simulink model "gravcomp"  (Simulink 7.5)
settings: Solver=ode3  StartTime=0.0  StopTime=inf  FixedStep=.002  RelTol=1e-3
undefined symbols (not defined in the file or in its folder): arm_home, arm_j2mt, arm_m2jp, bit, CAN_init, enc_per_rev, fdesignblkfcn, FT_init, gcbh, hand_on, MT_init, puck_I_per_Nm, rotFT2Hand, sample_time, Standard, VL1_init, VL2_init
libraries: simulink x358, xpclib x28, xpcutilitieslib x6, dspmathops x1
(part 3 of 3)

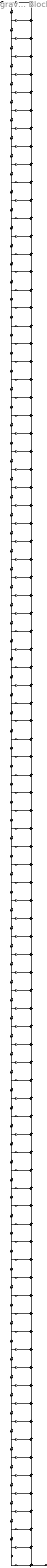
== system gravcomp/Get FT/Get Force Torque/Original Filter/Generated Filter Block ==
  Input : Inport
  BodyDelay{2..88} (87 alike) : simulink/Discrete/Integer Delay  vinit=0  samptime=-1  NumDelays=1
  BodyLSum{2..88} (87 alike) : Sum  Inputs=++|  OutScaling=1  RndMeth=Nearest  SaturateOnIntegerOverflow=on  OutDataTypeStr=Inherit: Same as first input
  b(1) : Gain  Gain=0.00082134311329855878  ParameterDataTypeMode=Specify via dialog  ParameterDataType=float('double')  ParamDataTypeStr=float('double')  OutScaling=1  RndMeth=Nearest  SaturateOnIntegerOverflow=on  OutDataTypeStr=Inherit: Same as input
  b(10) : Gain  Gain=-0.0024150838129607284  ParameterDataTypeMode=Specify via dialog  ParameterDataType=float('double')  ParamDataTypeStr=float('double')  OutScaling=1  RndMeth=Nearest  SaturateOnIntegerOverflow=on  OutDataTypeStr=Inherit: Same as input
  b(11) : Gain  Gain=-0.0039600576183871855  ParameterDataTypeMode=Specify via dialog  ParameterDataType=float('double')  ParamDataTypeStr=float('double')  OutScaling=1  RndMeth=Nearest  SaturateOnIntegerOverflow=on  OutDataTypeStr=Inherit: Same as input
  b(12) : Gain  Gain=-0.0054879111338127914  ParameterDataTypeMode=Specify via dialog  ParameterDataType=float('double')  ParamDataTypeStr=float('double')  OutScaling=1  RndMeth=Nearest  SaturateOnIntegerOverflow=on  OutDataTypeStr=Inherit: Same as input
  b(13) : Gain  Gain=-0.006789571651036521  ParameterDataTypeMode=Specify via dialog  ParameterDataType=float('double')  ParamDataTypeStr=float('double')  OutScaling=1  RndMeth=Nearest  SaturateOnIntegerOverflow=on  OutDataTypeStr=Inherit: Same as input
  b(14) : Gain  Gain=-0.007643017635847205  ParameterDataTypeMode=Specify via dialog  ParameterDataType=float('double')  ParamDataTypeStr=float('double')  OutScaling=1  RndMeth=Nearest  SaturateOnIntegerOverflow=on  OutDataTypeStr=Inherit: Same as input
  b(15) : Gain  Gain=-0.0078436359305586525  ParameterDataTypeMode=Specify via dialog  ParameterDataType=float('double')  ParamDataTypeStr=float('double')  OutScaling=1  RndMeth=Nearest  SaturateOnIntegerOverflow=on  OutDataTypeStr=Inherit: Same as input
  b(16) : Gain  Gain=-0.0072403435516525706  ParameterDataTypeMode=Specify via dialog  ParameterDataType=float('double')  ParamDataTypeStr=float('double')  OutScaling=1  RndMeth=Nearest  SaturateOnIntegerOverflow=on  OutDataTypeStr=Inherit: Same as input
  b(17) : Gain  Gain=-0.0057673738553609957  ParameterDataTypeMode=Specify via dialog  ParameterDataType=float('double')  ParamDataTypeStr=float('double')  OutScaling=1  RndMeth=Nearest  SaturateOnIntegerOverflow=on  OutDataTypeStr=Inherit: Same as input
  b(18) : Gain  Gain=-0.0034717942727364942  ParameterDataTypeMode=Specify via dialog  ParameterDataType=float('double')  ParamDataTypeStr=float('double')  OutScaling=1  RndMeth=Nearest  SaturateOnIntegerOverflow=on  OutDataTypeStr=Inherit: Same as input
  b(19) : Gain  Gain=-0.00052673802500832409  ParameterDataTypeMode=Specify via dialog  ParameterDataType=float('double')  ParamDataTypeStr=float('double')  OutScaling=1  RndMeth=Nearest  SaturateOnIntegerOverflow=on  OutDataTypeStr=Inherit: Same as input
  b(2) : Gain  Gain=0.00086044183774138872  ParameterDataTypeMode=Specify via dialog  ParameterDataType=float('double')  ParamDataTypeStr=float('double')  OutScaling=1  RndMeth=Nearest  SaturateOnIntegerOverflow=on  OutDataTypeStr=Inherit: Same as input
  b(20) : Gain  Gain=0.0027718950549306624  ParameterDataTypeMode=Specify via dialog  ParameterDataType=float('double')  ParamDataTypeStr=float('double')  OutScaling=1  RndMeth=Nearest  SaturateOnIntegerOverflow=on  OutDataTypeStr=Inherit: Same as input
  b(21) : Gain  Gain=0.0060277239934803696  ParameterDataTypeMode=Specify via dialog  ParameterDataType=float('double')  ParamDataTypeStr=float('double')  OutScaling=1  RndMeth=Nearest  SaturateOnIntegerOverflow=on  OutDataTypeStr=Inherit: Same as input
  b(22) : Gain  Gain=0.008783844113631022  ParameterDataTypeMode=Specify via dialog  ParameterDataType=float('double')  ParamDataTypeStr=float('double')  OutScaling=1  RndMeth=Nearest  SaturateOnIntegerOverflow=on  OutDataTypeStr=Inherit: Same as input
  b(23) : Gain  Gain=0.010579384955155813  ParameterDataTypeMode=Specify via dialog  ParameterDataType=float('double')  ParamDataTypeStr=float('double')  OutScaling=1  RndMeth=Nearest  SaturateOnIntegerOverflow=on  OutDataTypeStr=Inherit: Same as input
  b(24) : Gain  Gain=0.011014410167142509  ParameterDataTypeMode=Specify via dialog  ParameterDataType=float('double')  ParamDataTypeStr=float('double')  OutScaling=1  RndMeth=Nearest  SaturateOnIntegerOverflow=on  OutDataTypeStr=Inherit: Same as input
  b(25) : Gain  Gain=0.0098173087600081296  ParameterDataTypeMode=Specify via dialog  ParameterDataType=float('double')  ParamDataTypeStr=float('double')  OutScaling=1  RndMeth=Nearest  SaturateOnIntegerOverflow=on  OutDataTypeStr=Inherit: Same as input
  b(26) : Gain  Gain=0.006903687414337915  ParameterDataTypeMode=Specify via dialog  ParameterDataType=float('double')  ParamDataTypeStr=float('double')  OutScaling=1  RndMeth=Nearest  SaturateOnIntegerOverflow=on  OutDataTypeStr=Inherit: Same as input
  b(27) : Gain  Gain=0.0024180557419036216  ParameterDataTypeMode=Specify via dialog  ParameterDataType=float('double')  ParamDataTypeStr=float('double')  OutScaling=1  RndMeth=Nearest  SaturateOnIntegerOverflow=on  OutDataTypeStr=Inherit: Same as input
  b(28) : Gain  Gain=-0.0032497931384978924  ParameterDataTypeMode=Specify via dialog  ParameterDataType=float('double')  ParamDataTypeStr=float('double')  OutScaling=1  RndMeth=Nearest  SaturateOnIntegerOverflow=on  OutDataTypeStr=Inherit: Same as input
  b(29) : Gain  Gain=-0.0094784288355618199  ParameterDataTypeMode=Specify via dialog  ParameterDataType=float('double')  ParamDataTypeStr=float('double')  OutScaling=1  RndMeth=Nearest  SaturateOnIntegerOverflow=on  OutDataTypeStr=Inherit: Same as input
  b(3) : Gain  Gain=0.0011650777729447837  ParameterDataTypeMode=Specify via dialog  ParameterDataType=float('double')  ParamDataTypeStr=float('double')  OutScaling=1  RndMeth=Nearest  SaturateOnIntegerOverflow=on  OutDataTypeStr=Inherit: Same as input
  b(30) : Gain  Gain=-0.015461211888206202  ParameterDataTypeMode=Specify via dialog  ParameterDataType=float('double')  ParamDataTypeStr=float('double')  OutScaling=1  RndMeth=Nearest  SaturateOnIntegerOverflow=on  OutDataTypeStr=Inherit: Same as input
  b(31) : Gain  Gain=-0.020281532807071435  ParameterDataTypeMode=Specify via dialog  ParameterDataType=float('double')  ParamDataTypeStr=float('double')  OutScaling=1  RndMeth=Nearest  SaturateOnIntegerOverflow=on  OutDataTypeStr=Inherit: Same as input
  b(32) : Gain  Gain=-0.023010985299838312  ParameterDataTypeMode=Specify via dialog  ParameterDataType=float('double')  ParamDataTypeStr=float('double')  OutScaling=1  RndMeth=Nearest  SaturateOnIntegerOverflow=on  OutDataTypeStr=Inherit: Same as input
  b(33) : Gain  Gain=-0.022819440668883396  ParameterDataTypeMode=Specify via dialog  ParameterDataType=float('double')  ParamDataTypeStr=float('double')  OutScaling=1  RndMeth=Nearest  SaturateOnIntegerOverflow=on  OutDataTypeStr=Inherit: Same as input
  b(34) : Gain  Gain=-0.01908434796516191  ParameterDataTypeMode=Specify via dialog  ParameterDataType=float('double')  ParamDataTypeStr=float('double')  OutScaling=1  RndMeth=Nearest  SaturateOnIntegerOverflow=on  OutDataTypeStr=Inherit: Same as input
  b(35) : Gain  Gain=-0.011485203310779294  ParameterDataTypeMode=Specify via dialog  ParameterDataType=float('double')  ParamDataTypeStr=float('double')  OutScaling=1  RndMeth=Nearest  SaturateOnIntegerOverflow=on  OutDataTypeStr=Inherit: Same as input
  b(36) : Gain  Gain=-7.045886460328981e-005  ParameterDataTypeMode=Specify via dialog  ParameterDataType=float('double')  ParamDataTypeStr=float('double')  OutScaling=1  RndMeth=Nearest  SaturateOnIntegerOverflow=on  OutDataTypeStr=Inherit: Same as input
  b(37) : Gain  Gain=0.0147140504913441  ParameterDataTypeMode=Specify via dialog  ParameterDataType=float('double')  ParamDataTypeStr=float('double')  OutScaling=1  RndMeth=Nearest  SaturateOnIntegerOverflow=on  OutDataTypeStr=Inherit: Same as input
  b(38) : Gain  Gain=0.032040450344852957  ParameterDataTypeMode=Specify via dialog  ParameterDataType=float('double')  ParamDataTypeStr=float('double')  OutScaling=1  RndMeth=Nearest  SaturateOnIntegerOverflow=on  OutDataTypeStr=Inherit: Same as input
  b(39) : Gain  Gain=0.050759005066959656  ParameterDataTypeMode=Specify via dialog  ParameterDataType=float('double')  ParamDataTypeStr=float('double')  OutScaling=1  RndMeth=Nearest  SaturateOnIntegerOverflow=on  OutDataTypeStr=Inherit: Same as input
  b(4) : Gain  Gain=0.0013989605197153431  ParameterDataTypeMode=Specify via dialog  ParameterDataType=float('double')  ParamDataTypeStr=float('double')  OutScaling=1  RndMeth=Nearest  SaturateOnIntegerOverflow=on  OutDataTypeStr=Inherit: Same as input
  b(40) : Gain  Gain=0.069498089116120501  ParameterDataTypeMode=Specify via dialog  ParameterDataType=float('double')  ParamDataTypeStr=float('double')  OutScaling=1  RndMeth=Nearest  SaturateOnIntegerOverflow=on  OutDataTypeStr=Inherit: Same as input
  b(41) : Gain  Gain=0.086794001009398575  ParameterDataTypeMode=Specify via dialog  ParameterDataType=float('double')  ParamDataTypeStr=float('double')  OutScaling=1  RndMeth=Nearest  SaturateOnIntegerOverflow=on  OutDataTypeStr=Inherit: Same as input
  b(42) : Gain  Gain=0.10123636540766748  ParameterDataTypeMode=Specify via dialog  ParameterDataType=float('double')  ParamDataTypeStr=float('double')  OutScaling=1  RndMeth=Nearest  SaturateOnIntegerOverflow=on  OutDataTypeStr=Inherit: Same as input
  b(43) : Gain  Gain=0.11161274108764474  ParameterDataTypeMode=Specify via dialog  ParameterDataType=float('double')  ParamDataTypeStr=float('double')  OutScaling=1  RndMeth=Nearest  SaturateOnIntegerOverflow=on  OutDataTypeStr=Inherit: Same as input
  b(44) : Gain  Gain=0.11703538988284418  ParameterDataTypeMode=Specify via dialog  ParameterDataType=float('double')  ParamDataTypeStr=float('double')  OutScaling=1  RndMeth=Nearest  SaturateOnIntegerOverflow=on  OutDataTypeStr=Inherit: Same as input
  b(45) : Gain  Gain=0.11703538988284418  ParameterDataTypeMode=Specify via dialog  ParameterDataType=float('double')  ParamDataTypeStr=float('double')  OutScaling=1  RndMeth=Nearest  SaturateOnIntegerOverflow=on  OutDataTypeStr=Inherit: Same as input
  b(46) : Gain  Gain=0.11161274108764474  ParameterDataTypeMode=Specify via dialog  ParameterDataType=float('double')  ParamDataTypeStr=float('double')  OutScaling=1  RndMeth=Nearest  SaturateOnIntegerOverflow=on  OutDataTypeStr=Inherit: Same as input
  b(47) : Gain  Gain=0.10123636540766748  ParameterDataTypeMode=Specify via dialog  ParameterDataType=float('double')  ParamDataTypeStr=float('double')  OutScaling=1  RndMeth=Nearest  SaturateOnIntegerOverflow=on  OutDataTypeStr=Inherit: Same as input
  b(48) : Gain  Gain=0.086794001009398575  ParameterDataTypeMode=Specify via dialog  ParameterDataType=float('double')  ParamDataTypeStr=float('double')  OutScaling=1  RndMeth=Nearest  SaturateOnIntegerOverflow=on  OutDataTypeStr=Inherit: Same as input
  b(49) : Gain  Gain=0.069498089116120501  ParameterDataTypeMode=Specify via dialog  ParameterDataType=float('double')  ParamDataTypeStr=float('double')  OutScaling=1  RndMeth=Nearest  SaturateOnIntegerOverflow=on  OutDataTypeStr=Inherit: Same as input
  b(5) : Gain  Gain=0.0014807379825975565  ParameterDataTypeMode=Specify via dialog  ParameterDataType=float('double')  ParamDataTypeStr=float('double')  OutScaling=1  RndMeth=Nearest  SaturateOnIntegerOverflow=on  OutDataTypeStr=Inherit: Same as input
  b(50) : Gain  Gain=0.050759005066959656  ParameterDataTypeMode=Specify via dialog  ParameterDataType=float('double')  ParamDataTypeStr=float('double')  OutScaling=1  RndMeth=Nearest  SaturateOnIntegerOverflow=on  OutDataTypeStr=Inherit: Same as input
  b(51) : Gain  Gain=0.032040450344852957  ParameterDataTypeMode=Specify via dialog  ParameterDataType=float('double')  ParamDataTypeStr=float('double')  OutScaling=1  RndMeth=Nearest  SaturateOnIntegerOverflow=on  OutDataTypeStr=Inherit: Same as input
  b(52) : Gain  Gain=0.0147140504913441  ParameterDataTypeMode=Specify via dialog  ParameterDataType=float('double')  ParamDataTypeStr=float('double')  OutScaling=1  RndMeth=Nearest  SaturateOnIntegerOverflow=on  OutDataTypeStr=Inherit: Same as input
  b(53) : Gain  Gain=-7.045886460328981e-005  ParameterDataTypeMode=Specify via dialog  ParameterDataType=float('double')  ParamDataTypeStr=float('double')  OutScaling=1  RndMeth=Nearest  SaturateOnIntegerOverflow=on  OutDataTypeStr=Inherit: Same as input
  b(54) : Gain  Gain=-0.011485203310779294  ParameterDataTypeMode=Specify via dialog  ParameterDataType=float('double')  ParamDataTypeStr=float('double')  OutScaling=1  RndMeth=Nearest  SaturateOnIntegerOverflow=on  OutDataTypeStr=Inherit: Same as input
  b(55) : Gain  Gain=-0.01908434796516191  ParameterDataTypeMode=Specify via dialog  ParameterDataType=float('double')  ParamDataTypeStr=float('double')  OutScaling=1  RndMeth=Nearest  SaturateOnIntegerOverflow=on  OutDataTypeStr=Inherit: Same as input
  b(56) : Gain  Gain=-0.022819440668883396  ParameterDataTypeMode=Specify via dialog  ParameterDataType=float('double')  ParamDataTypeStr=float('double')  OutScaling=1  RndMeth=Nearest  SaturateOnIntegerOverflow=on  OutDataTypeStr=Inherit: Same as input
  b(57) : Gain  Gain=-0.023010985299838312  ParameterDataTypeMode=Specify via dialog  ParameterDataType=float('double')  ParamDataTypeStr=float('double')  OutScaling=1  RndMeth=Nearest  SaturateOnIntegerOverflow=on  OutDataTypeStr=Inherit: Same as input
  b(58) : Gain  Gain=-0.020281532807071435  ParameterDataTypeMode=Specify via dialog  ParameterDataType=float('double')  ParamDataTypeStr=float('double')  OutScaling=1  RndMeth=Nearest  SaturateOnIntegerOverflow=on  OutDataTypeStr=Inherit: Same as input
  b(59) : Gain  Gain=-0.015461211888206202  ParameterDataTypeMode=Specify via dialog  ParameterDataType=float('double')  ParamDataTypeStr=float('double')  OutScaling=1  RndMeth=Nearest  SaturateOnIntegerOverflow=on  OutDataTypeStr=Inherit: Same as input
  b(6) : Gain  Gain=0.0013305171923252142  ParameterDataTypeMode=Specify via dialog  ParameterDataType=float('double')  ParamDataTypeStr=float('double')  OutScaling=1  RndMeth=Nearest  SaturateOnIntegerOverflow=on  OutDataTypeStr=Inherit: Same as input
  b(60) : Gain  Gain=-0.0094784288355618199  ParameterDataTypeMode=Specify via dialog  ParameterDataType=float('double')  ParamDataTypeStr=float('double')  OutScaling=1  RndMeth=Nearest  SaturateOnIntegerOverflow=on  OutDataTypeStr=Inherit: Same as input
  b(61) : Gain  Gain=-0.0032497931384978924  ParameterDataTypeMode=Specify via dialog  ParameterDataType=float('double')  ParamDataTypeStr=float('double')  OutScaling=1  RndMeth=Nearest  SaturateOnIntegerOverflow=on  OutDataTypeStr=Inherit: Same as input
  b(62) : Gain  Gain=0.0024180557419036216  ParameterDataTypeMode=Specify via dialog  ParameterDataType=float('double')  ParamDataTypeStr=float('double')  OutScaling=1  RndMeth=Nearest  SaturateOnIntegerOverflow=on  OutDataTypeStr=Inherit: Same as input
  b(63) : Gain  Gain=0.006903687414337915  ParameterDataTypeMode=Specify via dialog  ParameterDataType=float('double')  ParamDataTypeStr=float('double')  OutScaling=1  RndMeth=Nearest  SaturateOnIntegerOverflow=on  OutDataTypeStr=Inherit: Same as input
  b(64) : Gain  Gain=0.0098173087600081296  ParameterDataTypeMode=Specify via dialog  ParameterDataType=float('double')  ParamDataTypeStr=float('double')  OutScaling=1  RndMeth=Nearest  SaturateOnIntegerOverflow=on  OutDataTypeStr=Inherit: Same as input
  b(65) : Gain  Gain=0.011014410167142509  ParameterDataTypeMode=Specify via dialog  ParameterDataType=float('double')  ParamDataTypeStr=float('double')  OutScaling=1  RndMeth=Nearest  SaturateOnIntegerOverflow=on  OutDataTypeStr=Inherit: Same as input
  b(66) : Gain  Gain=0.010579384955155813  ParameterDataTypeMode=Specify via dialog  ParameterDataType=float('double')  ParamDataTypeStr=float('double')  OutScaling=1  RndMeth=Nearest  SaturateOnIntegerOverflow=on  OutDataTypeStr=Inherit: Same as input
  b(67) : Gain  Gain=0.008783844113631022  ParameterDataTypeMode=Specify via dialog  ParameterDataType=float('double')  ParamDataTypeStr=float('double')  OutScaling=1  RndMeth=Nearest  SaturateOnIntegerOverflow=on  OutDataTypeStr=Inherit: Same as input
  b(68) : Gain  Gain=0.0060277239934803696  ParameterDataTypeMode=Specify via dialog  ParameterDataType=float('double')  ParamDataTypeStr=float('double')  OutScaling=1  RndMeth=Nearest  SaturateOnIntegerOverflow=on  OutDataTypeStr=Inherit: Same as input
  b(69) : Gain  Gain=0.0027718950549306624  ParameterDataTypeMode=Specify via dialog  ParameterDataType=float('double')  ParamDataTypeStr=float('double')  OutScaling=1  RndMeth=Nearest  SaturateOnIntegerOverflow=on  OutDataTypeStr=Inherit: Same as input
  b(7) : Gain  Gain=0.0008813799288182459  ParameterDataTypeMode=Specify via dialog  ParameterDataType=float('double')  ParamDataTypeStr=float('double')  OutScaling=1  RndMeth=Nearest  SaturateOnIntegerOverflow=on  OutDataTypeStr=Inherit: Same as input
  b(70) : Gain  Gain=-0.00052673802500832409  ParameterDataTypeMode=Specify via dialog  ParameterDataType=float('double')  ParamDataTypeStr=float('double')  OutScaling=1  RndMeth=Nearest  SaturateOnIntegerOverflow=on  OutDataTypeStr=Inherit: Same as input
  b(71) : Gain  Gain=-0.0034717942727364942  ParameterDataTypeMode=Specify via dialog  ParameterDataType=float('double')  ParamDataTypeStr=float('double')  OutScaling=1  RndMeth=Nearest  SaturateOnIntegerOverflow=on  OutDataTypeStr=Inherit: Same as input
  b(72) : Gain  Gain=-0.0057673738553609957  ParameterDataTypeMode=Specify via dialog  ParameterDataType=float('double')  ParamDataTypeStr=float('double')  OutScaling=1  RndMeth=Nearest  SaturateOnIntegerOverflow=on  OutDataTypeStr=Inherit: Same as input
  b(73) : Gain  Gain=-0.0072403435516525706  ParameterDataTypeMode=Specify via dialog  ParameterDataType=float('double')  ParamDataTypeStr=float('double')  OutScaling=1  RndMeth=Nearest  SaturateOnIntegerOverflow=on  OutDataTypeStr=Inherit: Same as input
  b(74) : Gain  Gain=-0.0078436359305586525  ParameterDataTypeMode=Specify via dialog  ParameterDataType=float('double')  ParamDataTypeStr=float('double')  OutScaling=1  RndMeth=Nearest  SaturateOnIntegerOverflow=on  OutDataTypeStr=Inherit: Same as input
  b(75) : Gain  Gain=-0.007643017635847205  ParameterDataTypeMode=Specify via dialog  ParameterDataType=float('double')  ParamDataTypeStr=float('double')  OutScaling=1  RndMeth=Nearest  SaturateOnIntegerOverflow=on  OutDataTypeStr=Inherit: Same as input
  b(76) : Gain  Gain=-0.006789571651036521  ParameterDataTypeMode=Specify via dialog  ParameterDataType=float('double')  ParamDataTypeStr=float('double')  OutScaling=1  RndMeth=Nearest  SaturateOnIntegerOverflow=on  OutDataTypeStr=Inherit: Same as input
  b(77) : Gain  Gain=-0.0054879111338127914  ParameterDataTypeMode=Specify via dialog  ParameterDataType=float('double')  ParamDataTypeStr=float('double')  OutScaling=1  RndMeth=Nearest  SaturateOnIntegerOverflow=on  OutDataTypeStr=Inherit: Same as input
  b(78) : Gain  Gain=-0.0039600576183871855  ParameterDataTypeMode=Specify via dialog  ParameterDataType=float('double')  ParamDataTypeStr=float('double')  OutScaling=1  RndMeth=Nearest  SaturateOnIntegerOverflow=on  OutDataTypeStr=Inherit: Same as input
  b(79) : Gain  Gain=-0.0024150838129607284  ParameterDataTypeMode=Specify via dialog  ParameterDataType=float('double')  ParamDataTypeStr=float('double')  OutScaling=1  RndMeth=Nearest  SaturateOnIntegerOverflow=on  OutDataTypeStr=Inherit: Same as input
  b(8) : Gain  Gain=9.3966665944649592e-005  ParameterDataTypeMode=Specify via dialog  ParameterDataType=float('double')  ParamDataTypeStr=float('double')  OutScaling=1  RndMeth=Nearest  SaturateOnIntegerOverflow=on  OutDataTypeStr=Inherit: Same as input
  b(80) : Gain  Gain=-0.0010242764933667812  ParameterDataTypeMode=Specify via dialog  ParameterDataType=float('double')  ParamDataTypeStr=float('double')  OutScaling=1  RndMeth=Nearest  SaturateOnIntegerOverflow=on  OutDataTypeStr=Inherit: Same as input
  b(81) : Gain  Gain=9.3966665944649592e-005  ParameterDataTypeMode=Specify via dialog  ParameterDataType=float('double')  ParamDataTypeStr=float('double')  OutScaling=1  RndMeth=Nearest  SaturateOnIntegerOverflow=on  OutDataTypeStr=Inherit: Same as input
  b(82) : Gain  Gain=0.0008813799288182459  ParameterDataTypeMode=Specify via dialog  ParameterDataType=float('double')  ParamDataTypeStr=float('double')  OutScaling=1  RndMeth=Nearest  SaturateOnIntegerOverflow=on  OutDataTypeStr=Inherit: Same as input
  b(83) : Gain  Gain=0.0013305171923252142  ParameterDataTypeMode=Specify via dialog  ParameterDataType=float('double')  ParamDataTypeStr=float('double')  OutScaling=1  RndMeth=Nearest  SaturateOnIntegerOverflow=on  OutDataTypeStr=Inherit: Same as input
  b(84) : Gain  Gain=0.0014807379825975565  ParameterDataTypeMode=Specify via dialog  ParameterDataType=float('double')  ParamDataTypeStr=float('double')  OutScaling=1  RndMeth=Nearest  SaturateOnIntegerOverflow=on  OutDataTypeStr=Inherit: Same as input
  b(85) : Gain  Gain=0.0013989605197153431  ParameterDataTypeMode=Specify via dialog  ParameterDataType=float('double')  ParamDataTypeStr=float('double')  OutScaling=1  RndMeth=Nearest  SaturateOnIntegerOverflow=on  OutDataTypeStr=Inherit: Same as input
  b(86) : Gain  Gain=0.0011650777729447837  ParameterDataTypeMode=Specify via dialog  ParameterDataType=float('double')  ParamDataTypeStr=float('double')  OutScaling=1  RndMeth=Nearest  SaturateOnIntegerOverflow=on  OutDataTypeStr=Inherit: Same as input
  b(87) : Gain  Gain=0.00086044183774138872  ParameterDataTypeMode=Specify via dialog  ParameterDataType=float('double')  ParamDataTypeStr=float('double')  OutScaling=1  RndMeth=Nearest  SaturateOnIntegerOverflow=on  OutDataTypeStr=Inherit: Same as input
  b(88) : Gain  Gain=0.00082134311329855878  ParameterDataTypeMode=Specify via dialog  ParameterDataType=float('double')  ParamDataTypeStr=float('double')  OutScaling=1  RndMeth=Nearest  SaturateOnIntegerOverflow=on  OutDataTypeStr=Inherit: Same as input
  b(9) : Gain  Gain=-0.0010242764933667812  ParameterDataTypeMode=Specify via dialog  ParameterDataType=float('double')  ParamDataTypeStr=float('double')  OutScaling=1  RndMeth=Nearest  SaturateOnIntegerOverflow=on  OutDataTypeStr=Inherit: Same as input
  Output : Outport
  wires:
  Input/1 -> b(1)/1, BodyDelay2/1
  b(1)/1 -> BodyLSum2/2
  BodyDelay2/1 -> b(2)/1, BodyDelay3/1
  b(2)/1 -> BodyLSum2/1
  BodyLSum2/1 -> BodyLSum3/2
  BodyDelay3/1 -> b(3)/1, BodyDelay4/1
  b(3)/1 -> BodyLSum3/1
  BodyLSum3/1 -> BodyLSum4/2
  BodyDelay4/1 -> b(4)/1, BodyDelay5/1
  b(4)/1 -> BodyLSum4/1
  BodyLSum4/1 -> BodyLSum5/2
  BodyDelay5/1 -> b(5)/1, BodyDelay6/1
  b(5)/1 -> BodyLSum5/1
  BodyLSum5/1 -> BodyLSum6/2
  BodyDelay6/1 -> b(6)/1, BodyDelay7/1
  b(6)/1 -> BodyLSum6/1
  BodyLSum6/1 -> BodyLSum7/2
  BodyDelay7/1 -> b(7)/1, BodyDelay8/1
  b(7)/1 -> BodyLSum7/1
  BodyLSum7/1 -> BodyLSum8/2
  BodyDelay8/1 -> b(8)/1, BodyDelay9/1
  b(8)/1 -> BodyLSum8/1
  BodyLSum8/1 -> BodyLSum9/2
  BodyDelay9/1 -> b(9)/1, BodyDelay10/1
  b(9)/1 -> BodyLSum9/1
  BodyLSum9/1 -> BodyLSum10/2
  BodyDelay10/1 -> b(10)/1, BodyDelay11/1
  b(10)/1 -> BodyLSum10/1
  BodyLSum10/1 -> BodyLSum11/2
  BodyDelay11/1 -> b(11)/1, BodyDelay12/1
  b(11)/1 -> BodyLSum11/1
  BodyLSum11/1 -> BodyLSum12/2
  BodyDelay12/1 -> b(12)/1, BodyDelay13/1
  b(12)/1 -> BodyLSum12/1
  BodyLSum12/1 -> BodyLSum13/2
  BodyDelay13/1 -> b(13)/1, BodyDelay14/1
  b(13)/1 -> BodyLSum13/1
  BodyLSum13/1 -> BodyLSum14/2
  BodyDelay14/1 -> b(14)/1, BodyDelay15/1
  b(14)/1 -> BodyLSum14/1
  BodyLSum14/1 -> BodyLSum15/2
  BodyDelay15/1 -> b(15)/1, BodyDelay16/1
  b(15)/1 -> BodyLSum15/1
  BodyLSum15/1 -> BodyLSum16/2
  BodyDelay16/1 -> b(16)/1, BodyDelay17/1
  b(16)/1 -> BodyLSum16/1
  BodyLSum16/1 -> BodyLSum17/2
  BodyDelay17/1 -> b(17)/1, BodyDelay18/1
  b(17)/1 -> BodyLSum17/1
  BodyLSum17/1 -> BodyLSum18/2
  BodyDelay18/1 -> b(18)/1, BodyDelay19/1
  b(18)/1 -> BodyLSum18/1
  BodyLSum18/1 -> BodyLSum19/2
  BodyDelay19/1 -> b(19)/1, BodyDelay20/1
  b(19)/1 -> BodyLSum19/1
  BodyLSum19/1 -> BodyLSum20/2
  BodyDelay20/1 -> b(20)/1, BodyDelay21/1
  b(20)/1 -> BodyLSum20/1
  BodyLSum20/1 -> BodyLSum21/2
  BodyDelay21/1 -> b(21)/1, BodyDelay22/1
  b(21)/1 -> BodyLSum21/1
  BodyLSum21/1 -> BodyLSum22/2
  BodyDelay22/1 -> b(22)/1, BodyDelay23/1
  b(22)/1 -> BodyLSum22/1
  BodyLSum22/1 -> BodyLSum23/2
  BodyDelay23/1 -> b(23)/1, BodyDelay24/1
  b(23)/1 -> BodyLSum23/1
  BodyLSum23/1 -> BodyLSum24/2
  BodyDelay24/1 -> b(24)/1, BodyDelay25/1
  b(24)/1 -> BodyLSum24/1
  BodyLSum24/1 -> BodyLSum25/2
  BodyDelay25/1 -> b(25)/1, BodyDelay26/1
  b(25)/1 -> BodyLSum25/1
  BodyLSum25/1 -> BodyLSum26/2
  BodyDelay26/1 -> b(26)/1, BodyDelay27/1
  b(26)/1 -> BodyLSum26/1
  BodyLSum26/1 -> BodyLSum27/2
  BodyDelay27/1 -> b(27)/1, BodyDelay28/1
  b(27)/1 -> BodyLSum27/1
  BodyLSum27/1 -> BodyLSum28/2
  BodyDelay28/1 -> b(28)/1, BodyDelay29/1
  b(28)/1 -> BodyLSum28/1
  BodyLSum28/1 -> BodyLSum29/2
  BodyDelay29/1 -> b(29)/1, BodyDelay30/1
  b(29)/1 -> BodyLSum29/1
  BodyLSum29/1 -> BodyLSum30/2
  BodyDelay30/1 -> b(30)/1, BodyDelay31/1
  b(30)/1 -> BodyLSum30/1
  BodyLSum30/1 -> BodyLSum31/2
  BodyDelay31/1 -> b(31)/1, BodyDelay32/1
  b(31)/1 -> BodyLSum31/1
  BodyLSum31/1 -> BodyLSum32/2
  BodyDelay32/1 -> b(32)/1, BodyDelay33/1
  b(32)/1 -> BodyLSum32/1
  BodyLSum32/1 -> BodyLSum33/2
  BodyDelay33/1 -> b(33)/1, BodyDelay34/1
  b(33)/1 -> BodyLSum33/1
  BodyLSum33/1 -> BodyLSum34/2
  BodyDelay34/1 -> b(34)/1, BodyDelay35/1
  b(34)/1 -> BodyLSum34/1
  BodyLSum34/1 -> BodyLSum35/2
  BodyDelay35/1 -> b(35)/1, BodyDelay36/1
  b(35)/1 -> BodyLSum35/1
  BodyLSum35/1 -> BodyLSum36/2
  BodyDelay36/1 -> b(36)/1, BodyDelay37/1
  b(36)/1 -> BodyLSum36/1
  BodyLSum36/1 -> BodyLSum37/2
  BodyDelay37/1 -> b(37)/1, BodyDelay38/1
  b(37)/1 -> BodyLSum37/1
  BodyLSum37/1 -> BodyLSum38/2
  BodyDelay38/1 -> b(38)/1, BodyDelay39/1
  b(38)/1 -> BodyLSum38/1
  BodyLSum38/1 -> BodyLSum39/2
  BodyDelay39/1 -> b(39)/1, BodyDelay40/1
  b(39)/1 -> BodyLSum39/1
  BodyLSum39/1 -> BodyLSum40/2
  BodyDelay40/1 -> b(40)/1, BodyDelay41/1
  b(40)/1 -> BodyLSum40/1
  BodyLSum40/1 -> BodyLSum41/2
  BodyDelay41/1 -> b(41)/1, BodyDelay42/1
  b(41)/1 -> BodyLSum41/1
  BodyLSum41/1 -> BodyLSum42/2
  BodyDelay42/1 -> b(42)/1, BodyDelay43/1
  b(42)/1 -> BodyLSum42/1
  BodyLSum42/1 -> BodyLSum43/2
  BodyDelay43/1 -> b(43)/1, BodyDelay44/1
  b(43)/1 -> BodyLSum43/1
  BodyLSum43/1 -> BodyLSum44/2
  BodyDelay44/1 -> b(44)/1, BodyDelay45/1
  b(44)/1 -> BodyLSum44/1
  BodyLSum44/1 -> BodyLSum45/2
  BodyDelay45/1 -> b(45)/1, BodyDelay46/1
  b(45)/1 -> BodyLSum45/1
  BodyLSum45/1 -> BodyLSum46/2
  BodyDelay46/1 -> b(46)/1, BodyDelay47/1
  b(46)/1 -> BodyLSum46/1
  BodyLSum46/1 -> BodyLSum47/2
  BodyDelay47/1 -> b(47)/1, BodyDelay48/1
  b(47)/1 -> BodyLSum47/1
  BodyLSum47/1 -> BodyLSum48/2
  BodyDelay48/1 -> b(48)/1, BodyDelay49/1
  b(48)/1 -> BodyLSum48/1
  BodyLSum48/1 -> BodyLSum49/2
  BodyDelay49/1 -> b(49)/1, BodyDelay50/1
  b(49)/1 -> BodyLSum49/1
  BodyLSum49/1 -> BodyLSum50/2
  BodyDelay50/1 -> b(50)/1, BodyDelay51/1
  b(50)/1 -> BodyLSum50/1
  BodyLSum50/1 -> BodyLSum51/2
  BodyDelay51/1 -> b(51)/1, BodyDelay52/1
  b(51)/1 -> BodyLSum51/1
  BodyLSum51/1 -> BodyLSum52/2
  BodyDelay52/1 -> b(52)/1, BodyDelay53/1
  b(52)/1 -> BodyLSum52/1
  BodyLSum52/1 -> BodyLSum53/2
  BodyDelay53/1 -> b(53)/1, BodyDelay54/1
  b(53)/1 -> BodyLSum53/1
  BodyLSum53/1 -> BodyLSum54/2
  BodyDelay54/1 -> b(54)/1, BodyDelay55/1
  b(54)/1 -> BodyLSum54/1
  BodyLSum54/1 -> BodyLSum55/2
  BodyDelay55/1 -> b(55)/1, BodyDelay56/1
  b(55)/1 -> BodyLSum55/1
  BodyLSum55/1 -> BodyLSum56/2
  BodyDelay56/1 -> b(56)/1, BodyDelay57/1
  b(56)/1 -> BodyLSum56/1
  BodyLSum56/1 -> BodyLSum57/2
  BodyDelay57/1 -> b(57)/1, BodyDelay58/1
  b(57)/1 -> BodyLSum57/1
  BodyLSum57/1 -> BodyLSum58/2
  BodyDelay58/1 -> b(58)/1, BodyDelay59/1
  b(58)/1 -> BodyLSum58/1
  BodyLSum58/1 -> BodyLSum59/2
  BodyDelay59/1 -> b(59)/1, BodyDelay60/1
  b(59)/1 -> BodyLSum59/1
  BodyLSum59/1 -> BodyLSum60/2
  BodyDelay60/1 -> b(60)/1, BodyDelay61/1
  b(60)/1 -> BodyLSum60/1
  BodyLSum60/1 -> BodyLSum61/2
  BodyDelay61/1 -> b(61)/1, BodyDelay62/1
  b(61)/1 -> BodyLSum61/1
  BodyLSum61/1 -> BodyLSum62/2
  BodyDelay62/1 -> b(62)/1, BodyDelay63/1
  b(62)/1 -> BodyLSum62/1
  BodyLSum62/1 -> BodyLSum63/2
  BodyDelay63/1 -> b(63)/1, BodyDelay64/1
  b(63)/1 -> BodyLSum63/1
  BodyLSum63/1 -> BodyLSum64/2
  BodyDelay64/1 -> b(64)/1, BodyDelay65/1
  b(64)/1 -> BodyLSum64/1
  BodyLSum64/1 -> BodyLSum65/2
  BodyDelay65/1 -> b(65)/1, BodyDelay66/1
  b(65)/1 -> BodyLSum65/1
  BodyLSum65/1 -> BodyLSum66/2
  BodyDelay66/1 -> b(66)/1, BodyDelay67/1
  b(66)/1 -> BodyLSum66/1
  BodyLSum66/1 -> BodyLSum67/2
  BodyDelay67/1 -> b(67)/1, BodyDelay68/1
  b(67)/1 -> BodyLSum67/1
  BodyLSum67/1 -> BodyLSum68/2
  BodyDelay68/1 -> b(68)/1, BodyDelay69/1
  b(68)/1 -> BodyLSum68/1
  BodyLSum68/1 -> BodyLSum69/2
  BodyDelay69/1 -> b(69)/1, BodyDelay70/1
  b(69)/1 -> BodyLSum69/1
  BodyLSum69/1 -> BodyLSum70/2
  BodyDelay70/1 -> b(70)/1, BodyDelay71/1
  b(70)/1 -> BodyLSum70/1
  BodyLSum70/1 -> BodyLSum71/2
  BodyDelay71/1 -> b(71)/1, BodyDelay72/1
  b(71)/1 -> BodyLSum71/1
  BodyLSum71/1 -> BodyLSum72/2
  BodyDelay72/1 -> b(72)/1, BodyDelay73/1
  b(72)/1 -> BodyLSum72/1
  BodyLSum72/1 -> BodyLSum73/2
  BodyDelay73/1 -> b(73)/1, BodyDelay74/1
  b(73)/1 -> BodyLSum73/1
  BodyLSum73/1 -> BodyLSum74/2
  BodyDelay74/1 -> b(74)/1, BodyDelay75/1
  b(74)/1 -> BodyLSum74/1
  BodyLSum74/1 -> BodyLSum75/2
  BodyDelay75/1 -> b(75)/1, BodyDelay76/1
  b(75)/1 -> BodyLSum75/1
  BodyLSum75/1 -> BodyLSum76/2
  BodyDelay76/1 -> b(76)/1, BodyDelay77/1
  b(76)/1 -> BodyLSum76/1
  BodyLSum76/1 -> BodyLSum77/2
  BodyDelay77/1 -> b(77)/1, BodyDelay78/1
  b(77)/1 -> BodyLSum77/1
  BodyLSum77/1 -> BodyLSum78/2
  BodyDelay78/1 -> b(78)/1, BodyDelay79/1
  b(78)/1 -> BodyLSum78/1
  BodyLSum78/1 -> BodyLSum79/2
  BodyDelay79/1 -> b(79)/1, BodyDelay80/1
  b(79)/1 -> BodyLSum79/1
  BodyLSum79/1 -> BodyLSum80/2
  BodyDelay80/1 -> b(80)/1, BodyDelay81/1
  b(80)/1 -> BodyLSum80/1
  BodyLSum80/1 -> BodyLSum81/2
  BodyDelay81/1 -> b(81)/1, BodyDelay82/1
  b(81)/1 -> BodyLSum81/1
  BodyLSum81/1 -> BodyLSum82/2
  BodyDelay82/1 -> b(82)/1, BodyDelay83/1
  b(82)/1 -> BodyLSum82/1
  BodyLSum82/1 -> BodyLSum83/2
  BodyDelay83/1 -> b(83)/1, BodyDelay84/1
  b(83)/1 -> BodyLSum83/1
  BodyLSum83/1 -> BodyLSum84/2
  BodyDelay84/1 -> b(84)/1, BodyDelay85/1
  b(84)/1 -> BodyLSum84/1
  BodyLSum84/1 -> BodyLSum85/2
  BodyDelay85/1 -> b(85)/1, BodyDelay86/1
  b(85)/1 -> BodyLSum85/1
  BodyLSum85/1 -> BodyLSum86/2
  BodyDelay86/1 -> b(86)/1, BodyDelay87/1
  b(86)/1 -> BodyLSum86/1
  BodyLSum86/1 -> BodyLSum87/2
  BodyDelay87/1 -> b(87)/1, BodyDelay88/1
  b(87)/1 -> BodyLSum87/1
  BodyLSum87/1 -> BodyLSum88/1
  BodyDelay88/1 -> b(88)/1
  b(88)/1 -> BodyLSum88/2
  BodyLSum88/1 -> Output/1

== matlab function Torque Control/Gravity Comp ==
  data: hand_on input double; q input double; tau output double
%
% gravComp7DOFNum Compute inverse dynamics via recursive Newton-Euler formulation
%
% Recursive Newton-Euler for standard Denavit-Hartenberg notation.
%

% Copyright (C) 1993-2011, by Peter I. Corke
%
% This file originally was part of The Robotics Toolbox for Matlab (RTB).
%
% http://www.petercorke.com

%
% Simplified from rne_dh for 7DOF WAM to compute only torque from gravity by Hans Vorsteveld
% Does not use structures from RTB, only the RNE algorithm
%

function tau = gravComp7DOF(hand_on,q)

%-------------------------------------------------------------------------------------
%   SETUP THE ARM
%-------------------------------------------------------------------------------------    
    DH_a = [0 0 0.045 -0.045 0 0 0];
    DH_d = [0 0 .55 0 0.3 0 0.061];
    DH_alpha = [-pi/2 pi/2 -pi/2 pi/2 -pi/2 pi/2 0];

    m = [8.3936 4.8487 1.7251 2.17266212 0.35655692 0.40915886 0.07548270];
    
    com = zeros(3,7);
    com(:,1) = [0.3506e-3, 132.6795e-3, 0.6286e-3];
    com(:,2) = [-0.2230e-3, -21.3924e-3, 13.3754e-3];
    com(:,3) = [-38.7565e-3, 217.9078e-3, 0.0252e-3];
    com(:,4) = [0.00553408,0.00006822,0.11927695];
    com(:,5) = [0.00005483,0.02886286,0.00148493];
    com(:,6) = [-0.00005923,-0.01686123,0.02419052];
    com(:,7) = [ 0.00014836,0.00007252,-0.00335185];
    
    if hand_on
        %hand_mass = 1.3731;  %for Schunk Gripper
        %DH_d(7) = DH_d(7) + .0953; % Adding the distance to the hand frame for Schunk Gripper
        %com(:,7) = ([0.001127;	-0.000211;	0.054851].*hand_mass + com(:,7).*m(7))/(hand_mass + m(7)); % Finding the combined center of mass
        
        % For wooden 'foot'
        hand_mass = .254;   
        hand_mass = -.5;
        DH_d(7) = DH_d(7) + 0.095;
        com(:,7) = ([0;	0;	0.06].*hand_mass + com(:,7).*m(7))/(hand_mass + m(7)); % Finding the combined center of mass
        
        m(7) = m(7) + hand_mass; % Adding the mass of the hand
    end
%-------------------------------------------------------------------------------------
%  END SETUP OF THE ARM
%-------------------------------------------------------------------------------------
    
	z0 = [0;0;1];
    grav = [0 0 9.81];
	fext = zeros(6, 1);
    n = 7;
    
    tau = zeros(n,1);
    
    Fm = zeros(3,7);
    pstarm = zeros(3,7);
    Rm = zeros(3,3,7);
    vd = grav(:);

    %
    % init some variables, compute the link rotation matrices
    %
    for j=1:n,
        a = DH_a(j);
        d = DH_d(j);
        alpha = DH_alpha(j);
        Tj = getTransformDH(DH_a(j), d, alpha, q(j));
        
        pstar = [a; d*sin(alpha); d*cos(alpha)];
        if j == 1,
            pstar = eye(3) * pstar;
            Tj = eye(4) * Tj;
        end
        pstarm(:,j) = pstar;
        Rm(:,:,j) = Tj(1:3,1:3);
    end
    %
    %  the forward recursion
    %
    for j=1:n,
        Rt = Rm(:,:,j)';
        % revolute axis
        vd = Rt*vd;
        
        vhat = vd;
        F = m(j)*vhat;
        Fm(:,j) = F;
    end

    %
    %  the backward recursion
    %

    fext = fext(:);
    f = fext(1:3);		% force/moments on end of arm
    nn = fext(4:6);

    for j=n:-1:1,
        pstar = pstarm(:,j);

        if j == n,
            R = eye(3,3);
        else
            R = Rm(:,:,j+1);
        end
        r = com(:,j)';
        nn = R*(nn + cross(R'*pstar,f)) + ...
            cross(pstar+r',Fm(:,j));
        f = R*f + Fm(:,j);

        R = Rm(:,:,j);
        % revolute
        tau(j) = nn'*(R'*z0);
    end
end

function T = getTransformDH(a,d,alpha,q)
    ct = cos(q);
    st = sin(q);
    cb = cos(alpha);
    sb = sin(alpha);
    
    T = [ ct, -st*cb,  st*sb, a*ct;
          st,  ct*cb, -ct*sb, a*st;
          0, sb, cb, d;
          0, 0, 0, 1 ];
end

== matlab function Receive Controller Commands/Embedded MATLAB Function ==
  data: t input double; data input double; FTSIGNAL output double; rcvd input double; taredTime input double; taredTimeOut output double
function [FTSIGNAL, taredTimeOut]  = fcn(t,data, rcvd, taredTime)
%#eml
    
    tarenow = 0;
    biasFT = 0;
    readFT = 0;

    % If there is a new packet this cycle
    if(rcvd == 1)
        switch(data(1))  % Using a switch because we may want to implement other commands
            case 1 % Tare command
                tarenow = 1;
                taredTime = t;
        end
    else
        if(t == .002) % Just starting the model
            tarenow = 1;
            taredTime = t;
        end
    end
    
    % Must calculate bias from .5 seconds to 1.5 seconds after sending the tare command
    % More than 1.5 seconds, do not calculate bias
    if(t - taredTime > 1.5)
        biasFT = 0;
        readFT = 1;
    elseif(t - taredTime > .5)
        biasFT = 1;
        readFT = 1;
    end

    taredTimeOut = taredTime;
    FTSIGNAL = [tarenow biasFT readFT];
    
end

== matlab function Get FT/Calculate Static FT/StaticFT ==
  data: q input double; FTExp output double; hand_on input double
function FTExp = staticFT(q, hand_on)
%#eml

    FTExp = zeros(6,1);
    g = [0;0;-9.81]; % Gravity
    r = [0;0;0];

    % a, d, and alpha (b) DH parameters
    dh_a = [0 0 0.045 -0.045 0 0 0 0];
    dh_d = [0 0 0.55 0 0.3 0 .061 0]; % Not sure about dh_d(8) For the hand
    dh_b = [-pi/2 pi/2 -pi/2 pi/2 -pi/2 pi/2 0 0];
    
    % hand on
    if (hand_on)
        %dh_d(8) = 0.0953; % Schunk Gripper
        %r = [0.001127;	-0.000211;	0.054851];  % Distace to COM of hand in the F/T sensors frame
        %hand_mass = 1.3731;     % Mass in kg
        
        
        % For wooden 'foot'
        hand_mass = .254;   
        dh_d(8) = 0.095;
        r = [0;	0;	0.06];
    else
        hand_mass = 0;
        dh_d(8) = 0;
        r = [0;	0;	0.0];
    end
    
    % compute forward kinematics of initial position
    ct = cos([q; 0]);
    st = sin([q; 0]);
    cb = cos(dh_b);
    sb = sin(dh_b);        
    T0 = eye(4);
    for i=1:8
        T = [ ct(i), -st(i)*cb(i),  st(i)*sb(i), dh_a(i)*ct(i);
              st(i),  ct(i)*cb(i), -ct(i)*sb(i), dh_a(i)*st(i);
              0, sb(i), cb(i), dh_d(i);
              0, 0, 0, 1 ];
        T0 = T0*T;
    end
    
    R0Fg = T0(1:3,1:3)'*g;
    FTExp(1:3) = R0Fg*hand_mass;
    FTExp(4:6) = cross(r,FTExp(1:3));
    
    i = isnan(FTExp);
    FTExp(i) = 0;

end
